simulink model "rebuilt_model"  (R2013b)
settings: Solver=ode45  StartTime=0.0  StopTime=10.0  RelTol=1e-3
values from neighbouring files (symbols this model uses):
  d = 0.5    [rebuilt__model_vars.mat]
  df = 0.2    [rebuilt__model_vars.mat]
  k = 5    [rebuilt__model_vars.mat]
  kf = 2    [rebuilt__model_vars.mat]
  m = 1    [rebuilt__model_vars.mat]
undefined symbols (not defined in the file or in its folder): du
settings Model: Creator=JNB  LastModifiedBy=JNB

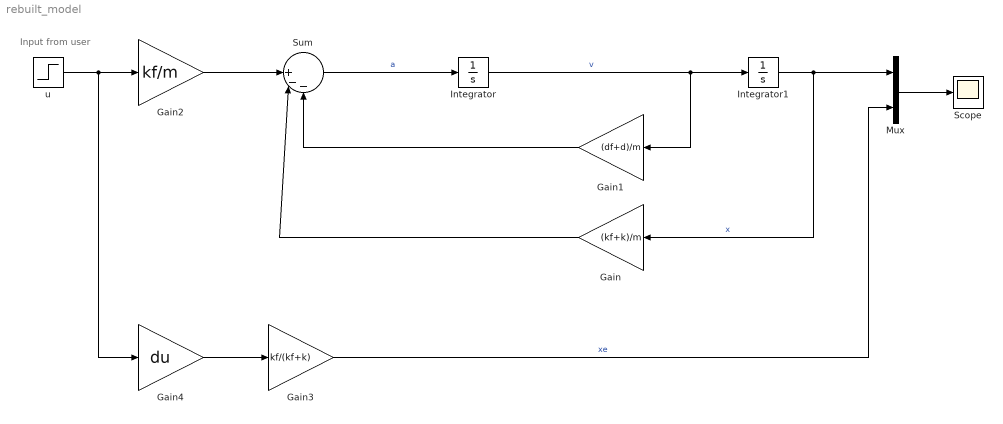
== system rebuilt_model ==
  note: Input from user
  Gain : Gain  Gain=(kf+k)/m
  Gain1 : Gain  Gain=(df+d)/m
  Gain2 : Gain  Gain=kf/m
  Gain3 : Gain  Gain=kf/(kf+k)
  Gain4 : Gain  Gain=du
  Integrator : Integrator
  Integrator1 : Integrator
  Mux : Mux  Inputs=2
  Scope : Scope
      settings: ShowLegends=on
  Sum : Sum  Inputs=||+--
  u : Step  SampleTime=0
  wires:
  Integrator/1 -> Gain1/1, Integrator1/1  "v"
  Integrator1/1 -> Mux/1, Gain/1  "x"
  Gain2/1 -> Sum/1
  Sum/1 -> Integrator/1  "a"
  Gain1/1 -> Sum/3
  Gain/1 -> Sum/2
  Mux/1 -> Scope/1
  u/1 -> Gain4/1, Gain2/1
  Gain4/1 -> Gain3/1
  Gain3/1 -> Mux/2  "xe"
